simulink model "lvbo_fangbo"  (R2020b)
settings: Solver=VariableStepAuto  StartTime=0.0  StopTime=0.005  RelTol=1e-3
libraries: dsparch4 x3
settings Model: Creator=QinKai  LastModifiedBy=QinKai

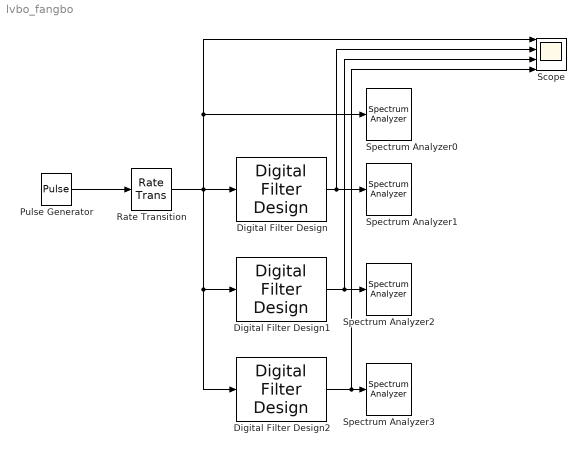
== system lvbo_fangbo ==
  Digital Filter Design : dsparch4/Digital Filter Design  mwdsp_browser_bugfix_var=off
  Digital Filter Design1 : dsparch4/Digital Filter Design  mwdsp_browser_bugfix_var=off
  Digital Filter Design2 : dsparch4/Digital Filter Design  mwdsp_browser_bugfix_var=off
  Pulse Generator : DiscretePulseGenerator  PulseType=Time based  Period=1/1e3  PulseWidth=50
  Rate Transition : RateTransition  OutPortSampleTime=1/20e3
  Scope : Scope  NumInputPorts=4
  Spectrum Analyzer{0..3} (4 alike) : SpectrumAnalyzer
  wires:
  Pulse Generator/1 -> Rate Transition/1
  Digital Filter Design/1 -> Scope/2, Spectrum Analyzer1/1
  Digital Filter Design1/1 -> Scope/3, Spectrum Analyzer2/1
  Digital Filter Design2/1 -> Scope/4, Spectrum Analyzer3/1
  Rate Transition/1 -> Digital Filter Design1/1, Digital Filter Design2/1, Digital Filter Design/1, Spectrum Analyzer0/1, Scope/1
